simulink model "benchmark_simani_generator_new"  (R2021b)
settings: Solver=VariableStepAuto  StartTime=0.0  StopTime=2000  RelTol=1e-1
values from neighbouring files (symbols this model uses):
  A = [ -B_dt/J B_dt/J -K_dt/J ... (first row only)    [benchmark_model_bianchi.m]    (also in benchmark_model_simani.m = [ -(B_dt+B_r)/J_r B_dt/N_g/J_r -K_dt/J_r)
  A_r = R_r^2 * pi    (= 10386.8907109)    [benchmark_model_bianchi.m]    (also in benchmark_model_simani.m)
  alpha_gc = 1/20e-3    (= 50)    [benchmark_model_bianchi.m]    (also in benchmark_model_simani.m)
  B = [1/J 0; 0 -1/J ; 0 0 ]    [benchmark_model_bianchi.m]    (also in benchmark_model_simani.m = [1/J_r 0; 0 -1/J_g ; 0 0 ])
  B_dt = 775.49    [benchmark_model_bianchi.m]    (also in benchmark_model_simani.m)
  C = [1 0 0; 0 1 0; 0 0 1]    [benchmark_model_bianchi.m]    (also in benchmark_model_simani.m = [1 0 0; 0 1/N_g 0; 0 0 1])
  cp_list = [0.0021 0.0031 0.0049 0.0065 0.0083 0.0127 0.0194 0.0344 0.0452 0.0693 0.0874 0.1129 ... (36 elements, 36x1)]    [bianchi.mat]    (also in simani.mat = [0.00196665 0.00290315 0.00458885 0.00608725 0.00777295 0.01)
  Cp_max = 0.4859    [benchmark_model_bianchi.m]    (also in benchmark_model_simani.m = 0.4554)
  eta_gc = 1    [benchmark_model_bianchi.m]    (also in benchmark_model_simani.m = 0.98)
  K_a = 0.5*rho_r*A_r    (= 6361.97056045)    [benchmark_model_bianchi.m]    (also in benchmark_model_simani.m)
  Kc = K_a*eta_dt*R_r^3*Cp_max/lambda_opt^3    (= 1147815.61138)    [benchmark_model_bianchi.m]    (also in benchmark_model_simani.m = 1043494.07808)
  omega_n = 11.11    [benchmark_model_bianchi.m]    (also in benchmark_model_simani.m)
  R_r = 57.5    [benchmark_model_bianchi.m]    (also in benchmark_model_simani.m)
  rho_r = 1.225    [benchmark_model_bianchi.m]    (also in benchmark_model_simani.m)
  v_0 = 7    [benchmark_model_bianchi.m]    (also in benchmark_model_simani.m)
  x0 = [omegar_0 omegag_0 (omegar_0-omegag_0)]    [benchmark_model_bianchi.m]    (also in benchmark_model_simani.m = [omegar_0 omegag_0 (omegar_0-omegag_0/N_g)])
  xi = 0.6    [benchmark_model_bianchi.m]    (also in benchmark_model_simani.m)
libraries: dspsrcs4 x3, spsWindTurbineLib x1
settings Model: Creator=spinolam  LastModifiedBy=manip
settings DebuggingCC: UnconnectedInputMsg=none  UnconnectedOutputMsg=none  UnconnectedLineMsg=none
settings RTWCC: DLArmComputeVersion=20.02.1

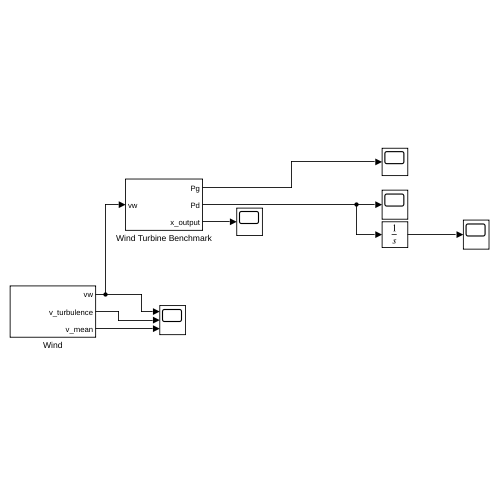
[thumbnail: Simulink's stored preview of the top-level diagram]
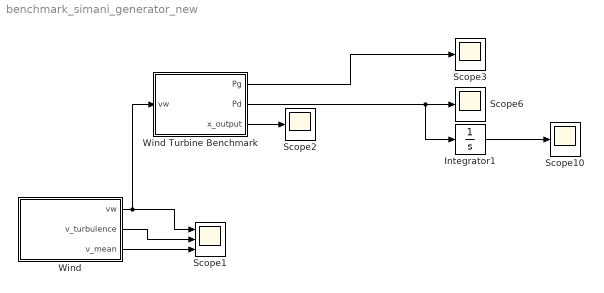
== system benchmark_simani_generator_new ==
  Integrator1 : Integrator
  Scope1 : Scope  NumInputPorts=3
  Scope{2..3,6,10} (4 alike) : Scope
  Wind : Subsystem
  Wind Turbine Benchmark : Subsystem
  wires:
  Wind Turbine Benchmark/1(Pg) -> Scope3/1
  Wind/1(vw) -> Scope1/1, Wind Turbine Benchmark/1(vw)
  Wind/2(v_turbulence) -> Scope1/2
  Wind Turbine Benchmark/2(Pd) -> Integrator1/1, Scope6/1
  Integrator1/1 -> Scope10/1
  Wind/3(v_mean) -> Scope1/3
  Wind Turbine Benchmark/3(x_output) -> Scope2/1

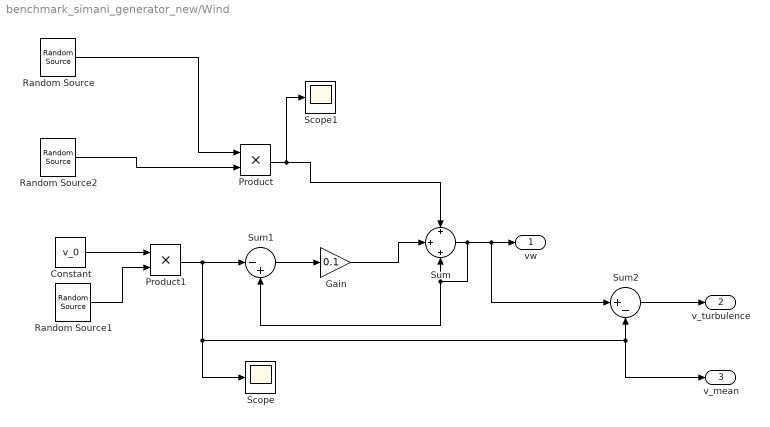
== system benchmark_simani_generator_new/Wind ==
  Constant : Constant  Value=v_0
  Gain : Gain  Gain=0.1
  Product : Product
  Product1 : Product
  Random Source : dspsrcs4/Random Source  SrcType=Gaussian  NormMethod=Ziggurat  CltLength=12  MinVal=0  MaxVal=0.5  MeanVal=0.03  VarVal=0.01  RepMode=Not repeatable  rawSeed=1  IsInherit=off  SampMode=Discrete  SampTime=10  SampFrame=1  DataType=Double  OutComplex=Real  OutputFrames=off
  Random Source1 : dspsrcs4/Random Source  SrcType=Gaussian  NormMethod=Ziggurat  CltLength=12  MinVal=0.8  MaxVal=1.2  MeanVal=1  VarVal=0.02  RepMode=Not repeatable  rawSeed=1  IsInherit=off  SampMode=Discrete  SampTime=60  SampFrame=1  DataType=Double  OutComplex=Real  OutputFrames=off
  Random Source2 : dspsrcs4/Random Source  SrcType=Uniform  NormMethod=Ziggurat  CltLength=12  MinVal=0  MaxVal=1  MeanVal=0.03  VarVal=0.01  RepMode=Not repeatable  rawSeed=1  IsInherit=off  SampMode=Discrete  SampTime=1  SampFrame=1  DataType=Double  OutComplex=Real  OutputFrames=off
  Scope : Scope
  Scope1 : Scope
  Sum : Sum  Inputs=+|+|+
  Sum1 : Sum  Inputs=|-+
  Sum2 : Sum  Inputs=|+-
  vw : Outport
  v_turbulence : Outport  Port=2
  v_mean : Outport  Port=3
  wires:
  Product1/1 -> Sum1/1, v_mean/1, Sum2/2, Scope/1
  Product/1 -> Sum/1, Scope1/1
  Gain/1 -> Sum/2
  Sum1/1 -> Gain/1
  Sum/1 -> Sum2/1, vw/1, Sum1/2, Sum/3
  Sum2/1 -> v_turbulence/1
  Random Source2/1 -> Product/2
  Random Source/1 -> Product/1
  Constant/1 -> Product1/1
  Random Source1/1 -> Product1/2

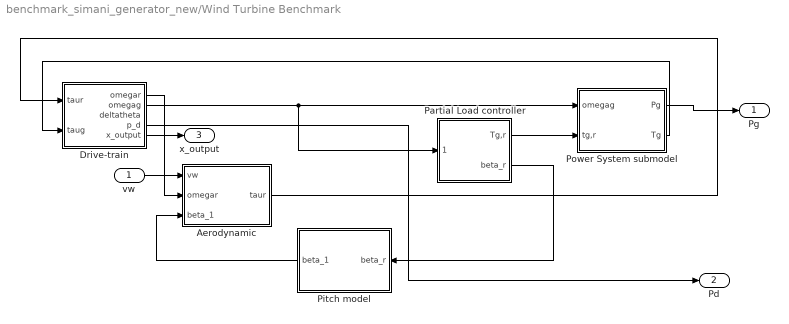
== system benchmark_simani_generator_new/Wind Turbine Benchmark ==
  vw : Inport
  Aerodynamic : Subsystem
  Drive-train : Subsystem
  Partial Load controller : Subsystem
  Pitch model : Subsystem
  Power System submodel : Subsystem
  Pg : Outport
  Pd : Outport  Port=2
  x_output : Outport  Port=3
  wires:
  Power System submodel/2(Tg) -> Drive-train/2(taug)
  Pitch model/1(beta_1) -> Aerodynamic/3(beta_1)
  Power System submodel/1(Pg) -> Pg/1
  Drive-train/1(omegar) -> Aerodynamic/2(omegar)
  Aerodynamic/1(taur) -> Drive-train/1(taur)
  Partial Load controller/2(beta_r) -> Pitch model/1(beta_r)
  Partial Load controller/1(Tg,r) -> Power System submodel/2(tg,r)
  vw/1 -> Aerodynamic/1(vw)
  Drive-train/4(p_d) -> Pd/1
  Drive-train/2(omegag) -> Partial Load controller/1(omegag), Power System submodel/1(omegag)
  Drive-train/5(x_output) -> x_output/1

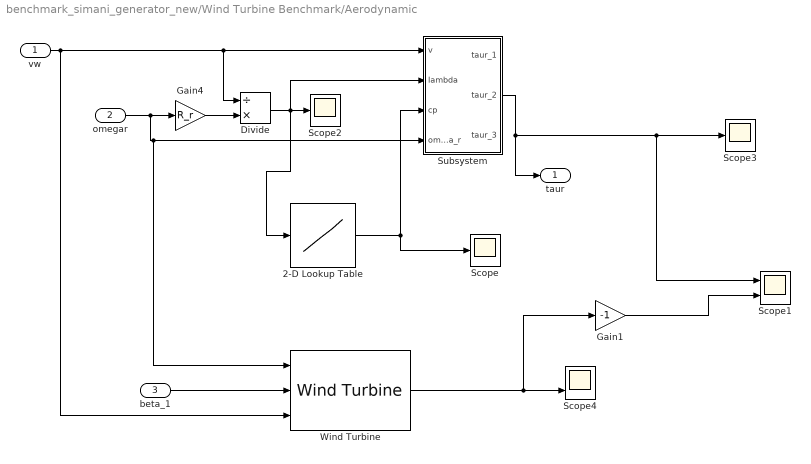
== system benchmark_simani_generator_new/Wind Turbine Benchmark/Aerodynamic ==
  vw : Inport
  omegar : Inport  Port=2
  beta_1 : Inport  Port=3
  2-D Lookup Table : Lookup_n-D  NumberOfTableDimensions=1  BreakpointsForDimension1=[0.411941585147336;0.599187760214307;0.878808714980984;1.09851089372623;1.31821307247148;1.64776634058934;1.88316153210211;2.19702178745246;2.35395191512763;2.63642614494295;2.82474229815316;3.07583050243344;3.29553268117869;3.59512656128584;3.8447881280418;4.11941585147336;4.39404357490492;4.5630452508628;4.83344793239541;5.07005027873644;5.2728522898859;5.57705530661009;5.7671821920627;6.08406033448373;6.59106536235738;7.09807039023102;7.41494853265205;7.90927843482885;8.3886286430003;8.78808714980984;9.52042774562732;10.3573884265616;11.2989691926126;12.2405499586637;13.1821307247148;15.3791525121672]  BreakpointsForDimension2=[0;1]  BreakpointsForDimension1DataTypeStr=Inherit: Inherit from 'Breakpoint data'  Table=cp_list  TableDataTypeStr=Inherit: Inherit from 'Table data'  InternalRulePriority=Speed  RndMeth=Simplest  InputSameDT=on
  Divide : Product  Inputs=/*
  Gain1 : Gain  Gain=-1
  Gain4 : Gain  Gain=R_r
  Scope : Scope
  Scope1 : Scope  NumInputPorts=2
  Scope2 : Scope
  Scope3 : Scope
  Scope4 : Scope  NumInputPorts=2
  Subsystem : Subsystem
  Wind Turbine : spsWindTurbineLib/Wind Turbine  Pnom=0.5*rho_r*A_r*v_0^3*Cp_max  Pelec_base=1  wind_base=v_0  P_wind_base=1  speed_nom=omegar_0  pitch_angle=0  c1_c6="[0.51763          116          0.4            5           21     0.006795]"  cp_nom=0.48  lambda_nom=8.1
      settings: SourceProductBaseCode=PS
  taur : Outport
  wires:
  2-D Lookup Table/1 -> Subsystem/3(cp), Scope/1
  vw/1 -> Wind Turbine/3, Subsystem/1(v), Divide/1
  omegar/1 -> Gain4/1, Wind Turbine/1, Subsystem/4(omega_r)
  Divide/1 -> Scope2/1, 2-D Lookup Table/1, Subsystem/2(Iambda)
  Subsystem/2(taur_2) -> Scope1/1, Scope3/1, taur/1
  Gain4/1 -> Divide/2
  beta_1/1 -> Wind Turbine/2
  Wind Turbine/1 -> Gain1/1, Scope4/2
  Gain1/1 -> Scope1/2

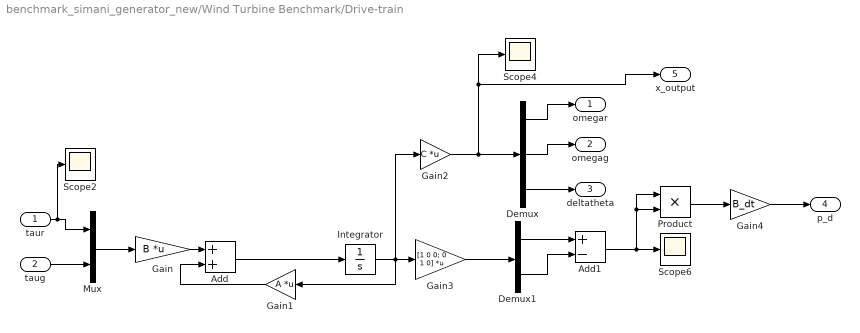
== system benchmark_simani_generator_new/Wind Turbine Benchmark/Drive-train ==
  taur : Inport
  taug : Inport  Port=2
  Add : Sum
  Add1 : Sum  Inputs=+-
  Demux : Demux  Outputs=3
  Demux1 : Demux  Outputs=2
  Gain : Gain  Gain=B  Multiplication=Matrix(K*u)
  Gain1 : Gain  Gain=A  Multiplication=Matrix(K*u)
  Gain2 : Gain  Gain=C  Multiplication=Matrix(K*u)
  Gain3 : Gain  Gain=[1 0 0; 0 1 0]  Multiplication=Matrix(K*u)
  Gain4 : Gain  Gain=B_dt
  Integrator : Integrator  InitialCondition=x0
  Mux : Mux  Inputs=2
  Product : Product
  Scope2 : Scope
  Scope4 : Scope
  Scope6 : Scope
  omegar : Outport
  omegag : Outport  Port=2
  deltatheta : Outport  Port=3
  p_d : Outport  Port=4
  x_output : Outport  Port=5
  wires:
  Integrator/1 -> Gain2/1, Gain1/1, Gain3/1
  Gain2/1 -> x_output/1, Scope4/1, Demux/1
  Add1/1 -> Product/1, Product/2, Scope6/1
  Demux/3 -> deltatheta/1
  Demux1/2 -> Add1/2
  Gain3/1 -> Demux1/1
  taur/1 -> Scope2/1, Mux/1
  taug/1 -> Mux/2
  Demux/1 -> omegar/1
  Gain4/1 -> p_d/1
  Mux/1 -> Gain/1
  Gain/1 -> Add/1
  Gain1/1 -> Add/2
  Add/1 -> Integrator/1
  Demux1/1 -> Add1/1
  Product/1 -> Gain4/1
  Demux/2 -> omegag/1

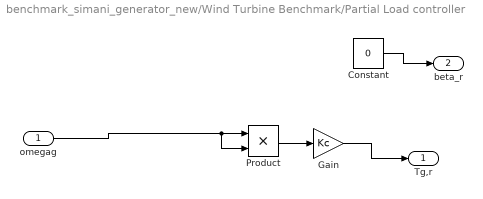
== system benchmark_simani_generator_new/Wind Turbine Benchmark/Partial Load controller ==
  omegag : Inport
  Constant : Constant  Value=0
  Gain : Gain  Gain=Kc
  Product : Product
  Tg,r : Outport
  beta_r : Outport  Port=2
  wires:
  Product/1 -> Gain/1
  Gain/1 -> Tg,r/1
  Constant/1 -> beta_r/1
  omegag/1 -> Product/2, Product/1

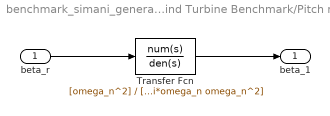
== system benchmark_simani_generator_new/Wind Turbine Benchmark/Pitch model ==
  beta_r : Inport
  Transfer Fcn : TransferFcn  Numerator=[omega_n^2]  Denominator=[1 2*xi*omega_n omega_n^2]
  beta_1 : Outport
  wires:
  beta_r/1 -> Transfer Fcn/1
  Transfer Fcn/1 -> beta_1/1

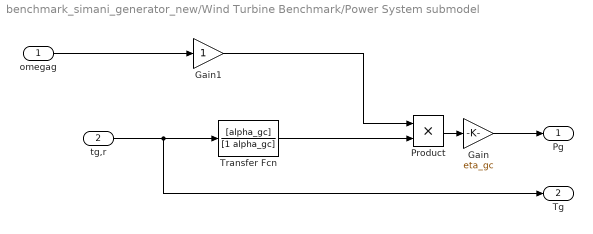
== system benchmark_simani_generator_new/Wind Turbine Benchmark/Power System submodel ==
  omegag : Inport
  tg,r : Inport  Port=2
  Gain : Gain  Gain=eta_gc
  Gain1 : Gain
  Product : Product
  Transfer Fcn : TransferFcn  Numerator=[alpha_gc]  Denominator=[1 alpha_gc]
  Pg : Outport
  Tg : Outport  Port=2
  wires:
  Product/1 -> Gain/1
  Gain/1 -> Pg/1
  omegag/1 -> Gain1/1
  tg,r/1 -> Tg/1, Transfer Fcn/1
  Transfer Fcn/1 -> Product/2
  Gain1/1 -> Product/1

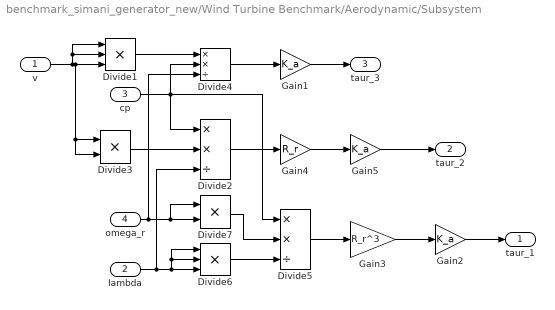
== system benchmark_simani_generator_new/Wind Turbine Benchmark/Aerodynamic/Subsystem ==
  v : Inport
  Iambda : Inport  Port=2
  cp : Inport  Port=3
  omega_r : Inport  Port=4
  Divide1 : Product  Inputs=***
  Divide2 : Product  Inputs=**/
  Divide3 : Product  Inputs=**
  Divide4 : Product  Inputs=**/
  Divide5 : Product  Inputs=**/
  Divide6 : Product  Inputs=***
  Divide7 : Product  Inputs=**
  Gain1 : Gain  Gain=K_a
  Gain2 : Gain  Gain=K_a
  Gain3 : Gain  Gain=R_r^3
  Gain4 : Gain  Gain=R_r
  Gain5 : Gain  Gain=K_a
  taur_1 : Outport
  taur_2 : Outport  Port=2
  taur_3 : Outport  Port=3
  wires:
  cp/1 -> Divide4/2, Divide5/1, Divide2/1
  Divide6/1 -> Divide5/3
  Divide2/1 -> Gain4/1
  Gain1/1 -> taur_3/1
  Divide1/1 -> Divide4/1
  Iambda/1 -> Divide6/2, Divide6/1, Divide6/3, Divide2/3
  Divide3/1 -> Divide2/2
  Gain5/1 -> taur_2/1
  Divide5/1 -> Gain3/1
  Divide7/1 -> Divide5/2
  Gain4/1 -> Gain5/1
  v/1 -> Divide3/1, Divide3/2, Divide1/3, Divide1/1, Divide1/2
  Divide4/1 -> Gain1/1
  Gain2/1 -> taur_1/1
  Gain3/1 -> Gain2/1
  omega_r/1 -> Divide7/1, Divide7/2, Divide4/3
